simulink model "PFC_69C_03_06_V01_3Phase_3_2KW"  (R2022b)
settings: Solver=FixedStepAuto  StartTime=0.0  StopTime=Inf  RelTol=1e-3  EnableMultiTasking=on
model workspace (MAT data in the model file):
  ADC_Gain = 1241.21212121
  DAC_Gain = 0.000805860805861
  Inductor_Current_Divider_Gain_Phase_A = 33.4
  Inductor_Current_Divider_Gain_Phase_B = 33.4
  Vbulk_Divider_Gain = 276.854928018
  Vin_Divider_Gain = 556.17352614
undefined symbols (not defined in the file or in its folder): GPTRIP1SEL, GPTRIP2SEL, SCI_A_Transmit, SCI_A_Transmit_Current_Suffix, SCI_A_Transmit_one_shot_Suffix, SCI_A_Transmit_Polarity_Suffix, SCI_A_Transmit_relay_Suffix, SCI_A_Transmit_Vbulk_Suffix, SCI_A_Transmit_Vin_rms_Suffix, SCI_A_Transmit_Vin_Suffix, SCI_A_Transmit_Vmid_Suffix, SCI_A_Transmit_Vp_Suffix, SCI_A_Transmit_Vpfc_Suffix, TZ1, TZ2
libraries: c280xlib x38, c2802xlib x34, simulink x17, c2000lib x1
(part 6 of 8)

== system PFC_69C_03_06_V01_3Phase_3_2KW/Calibration,RMS, Fault Protection @5kHz/Fault checking/If Action Subsystem/Phase_C_Fault ==
  function : TriggerPort  TriggerType=function-call  VariantControl=(inherit)
  Fault Check (Input OVP)_Phase_C : Subsystem  TreatAsAtomicUnit=on
  Fault Check (Input UVP)_Phase_C : Subsystem  TreatAsAtomicUnit=on
  Function-Call Generator : simulink/Ports & Subsystems/Function-Call Generator  sample_time=-1  numberOfIterations=1  DisallowWideOutput=off
  Function-Call Split : FunctionCallSplit  IconShape=distinctive  NumOutputPorts=3  OutputPortLayout=default
  Input current_OCP_Phase_C : Subsystem  TreatAsAtomicUnit=on
  wires:
  Function-Call Generator/1 -> Function-Call Split/1
  Function-Call Split/1 -> Fault Check (Input UVP)_Phase_C/Trigger
  Function-Call Split/2 -> Fault Check (Input OVP)_Phase_C/Trigger
  Function-Call Split/3 -> Input current_OCP_Phase_C/Trigger

== system PFC_69C_03_06_V01_3Phase_3_2KW/Calibration,RMS, Fault Protection @5kHz/Polarity & Near Zero check/Polarity_Near_zero_Phase_A/Volt to Number ==
  In1 : Inport
  Gain : Gain  Gain=ADC_Gain
  Gain1 : Gain  Gain=1/Vin_Divider_Gain
  Out1 : Outport
  wires:
  Gain1/1 -> Gain/1
  In1/1 -> Gain1/1
  Gain/1 -> Out1/1

== system PFC_69C_03_06_V01_3Phase_3_2KW/Calibration,RMS, Fault Protection @5kHz/Polarity & Near Zero check/Polarity_Near_zero_Phase_B/Volt to Number ==
  In1 : Inport
  Gain : Gain  Gain=ADC_Gain
  Gain1 : Gain  Gain=1/Vin_Divider_Gain
  Out1 : Outport
  wires:
  Gain1/1 -> Gain/1
  In1/1 -> Gain1/1
  Gain/1 -> Out1/1

== system PFC_69C_03_06_V01_3Phase_3_2KW/Calibration,RMS, Fault Protection @5kHz/Polarity & Near Zero check/Polarity_Near_zero_Phase_C/Volt to Number ==
  In1 : Inport
  Gain : Gain  Gain=ADC_Gain
  Gain1 : Gain  Gain=1/Vin_Divider_Gain
  Out1 : Outport
  wires:
  Gain1/1 -> Gain/1
  In1/1 -> Gain1/1
  Gain/1 -> Out1/1

== system PFC_69C_03_06_V01_3Phase_3_2KW/Calibration,RMS, Fault Protection @5kHz/Relay control/Subsystem/ADC Gain2 ==
  In1 : Inport
  Gain : Gain  Gain=ADC_Gain
  Gain1 : Gain  Gain=1/Vin_Divider_Gain
  Out1 : Outport
  wires:
  Gain1/1 -> Gain/1
  In1/1 -> Gain1/1
  Gain/1 -> Out1/1

== system PFC_69C_03_06_V01_3Phase_3_2KW/Calibration,RMS, Fault Protection @5kHz/Relay control/Subsystem/ADC Gain3 ==
  In1 : Inport
  Gain : Gain  Gain=ADC_Gain
  Gain1 : Gain  Gain=1/Vin_Divider_Gain
  Out1 : Outport
  wires:
  Gain1/1 -> Gain/1
  In1/1 -> Gain1/1
  Gain/1 -> Out1/1

== system PFC_69C_03_06_V01_3Phase_3_2KW/Calibration,RMS, Fault Protection @5kHz/Relay control_corrected/Subsystem/ADC Gain2 ==
  In1 : Inport
  Gain : Gain  Gain=ADC_Gain
  Gain1 : Gain  Gain=1/Vin_Divider_Gain
  Out1 : Outport
  wires:
  Gain1/1 -> Gain/1
  In1/1 -> Gain1/1
  Gain/1 -> Out1/1

== system PFC_69C_03_06_V01_3Phase_3_2KW/Calibration,RMS, Fault Protection @5kHz/Relay control_corrected/Subsystem/ADC Gain3 ==
  In1 : Inport
  Gain : Gain  Gain=ADC_Gain
  Gain1 : Gain  Gain=1/Vin_Divider_Gain
  Out1 : Outport
  wires:
  Gain1/1 -> Gain/1
  In1/1 -> Gain1/1
  Gain/1 -> Out1/1

== system PFC_69C_03_06_V01_3Phase_3_2KW/Calibration,RMS, Fault Protection @5kHz/Voltage RMS//Averag Calculation/Phase_A/RMS Current Calculation_Phase_A ==
  note: RMS Voltage Calculation
  function : TriggerPort  TriggerType=function-call  VariantControl=(inherit)
  Chart : Stateflow chart  TreatAsAtomicUnit=on
  Data Store Read2 : DataStoreRead  DataStoreName=Inductor_Current_ADC_Phase_A  IndexOptions=Index vector (dialog)  Indices=1  OutputSizes=1
  Data Store Read5 : DataStoreRead  DataStoreName=Inductor_Current_1_65_ADC_Phase_A  IndexOptions=Index vector (dialog)  Indices=1  OutputSizes=1
  Data Store Write : DataStoreWrite  DataStoreName=Iin_rms_Phase_A  IndexOptions=Index vector (dialog)  Indices=1  OutputSizes=1
  Data Store Write1 : DataStoreWrite  DataStoreName=Iin_peak_Phase_A  IndexOptions=Index vector (dialog)  Indices=1  OutputSizes=1
  Gain1 : Gain  Gain=DAC_Gain
  Gain2 : Gain  Gain=DAC_Gain
  Gain3 : Gain  Gain=Inductor_Current_Divider_Gain_Phase_B
  Gain4 : Gain  Gain=Inductor_Current_Divider_Gain_Phase_B
  Gain5 : Gain  Gain=100
  Gain6 : Gain  Gain=100
  Subtract2 : Sum  Inputs=+-
  wires:
  Data Store Read2/1 -> Subtract2/1
  Data Store Read5/1 -> Subtract2/2
  Subtract2/1 -> Chart/1(input)
  Gain2/1 -> Gain3/1
  Chart/2(Vrms) -> Gain2/1
  Gain3/1 -> Gain6/1
  Gain6/1 -> Data Store Write/1
  Gain4/1 -> Gain5/1
  Gain1/1 -> Gain4/1
  Chart/1(Vpeak) -> Gain1/1
  Gain5/1 -> Data Store Write1/1

== system PFC_69C_03_06_V01_3Phase_3_2KW/Calibration,RMS, Fault Protection @5kHz/Voltage RMS//Averag Calculation/Phase_A/RMS Voltage Calculation_Phase_A ==
  note: RMS Voltage Calculation
  function : TriggerPort  TriggerType=function-call  VariantControl=(inherit)
  Chart : Stateflow chart  TreatAsAtomicUnit=on
  Data Store Read2 : DataStoreRead  DataStoreName=Vin_ADC_Average_Phase_A  IndexOptions=Index vector (dialog)  Indices=1  OutputSizes=1
  Data Store Read5 : DataStoreRead  DataStoreName=Vin_1_65_ADC_Phase_A  IndexOptions=Index vector (dialog)  Indices=1  OutputSizes=1
  Data Store Write1 : DataStoreWrite  DataStoreName=Vin_peak_Phase_A  IndexOptions=Index vector (dialog)  Indices=1  OutputSizes=1
  Data Store Write2 : DataStoreWrite  DataStoreName=Vin_rms_Phase_A  IndexOptions=Index vector (dialog)  Indices=1  OutputSizes=1
  Data Store Write3 : DataStoreWrite  DataStoreName=Vin_peak_ADC_Phase_A  IndexOptions=Index vector (dialog)  Indices=1  OutputSizes=1
  Data Store Write4 : DataStoreWrite  DataStoreName=Vin_rms_ADC  IndexOptions=Index vector (dialog)  Indices=1  OutputSizes=1
  Digital Output : c280xlib/Digital Output  Commented=on  GPIO_Number=GPIO16~GPIO23  GPIO_Bit0=off  GPIO_BIT0_Toggle=off  GPIO_Bit1=off  GPIO_BIT1_Toggle=off  GPIO_Bit2=off  GPIO_BIT2_Toggle=off  GPIO_Bit3=off  GPIO_BIT3_Toggle=off  GPIO_Bit4=off  GPIO_BIT4_Toggle=off  GPIO_Bit5=off  GPIO_BIT5_Toggle=off  GPIO_Bit6=on  GPIO_BIT6_Toggle=off  GPIO_Bit7=off  GPIO_BIT7_Toggle=off
  Gain6 : Gain  Gain=DAC_Gain
  Gain7 : Gain  Gain=Vin_Divider_Gain  OutDataTypeStr=double
  Gain8 : Gain  Gain=DAC_Gain
  Gain9 : Gain  Gain=Vin_Divider_Gain  OutDataTypeStr=double
  Subtract2 : Sum  Inputs=+-
  wires:
  Chart/1(Vpeak) -> Data Store Write3/1, Gain8/1
  Chart/2(Vrms) -> Gain6/1, Data Store Write4/1
  Gain7/1 -> Data Store Write2/1
  Data Store Read2/1 -> Subtract2/1
  Gain8/1 -> Gain9/1
  Gain6/1 -> Gain7/1
  Data Store Read5/1 -> Subtract2/2
  Gain9/1 -> Data Store Write1/1
  Subtract2/1 -> Chart/1(input)

== system PFC_69C_03_06_V01_3Phase_3_2KW/Calibration,RMS, Fault Protection @5kHz/Voltage RMS//Averag Calculation/Phase_A/Vin_ADC Averaging_Phase_A ==
  note: Low pass filter :
      | 1kHz bandwidth with 5kHz switching freq
  function : TriggerPort  TriggerType=function-call  VariantControl=(inherit)
  Chart1 : Stateflow chart  TreatAsAtomicUnit=on
  Constant1 : Constant  Value=0.38586954
  Constant2 : Constant  Value=0.38586954
  Constant3 : Constant  Value=-0.22826091
  Data Store Read3 : DataStoreRead  DataStoreName=Vin_ADC_Phase_A  IndexOptions=Index vector (dialog)  Indices=1  OutputSizes=1
  Vin_ADC_Average : DataStoreWrite  DataStoreName=Vin_ADC_Average_Phase_A  IndexOptions=Index vector (dialog)  Indices=1  OutputSizes=1
  wires:
  Constant3/1 -> [a1]
  Constant1/1 -> [b0]
  Constant2/1 -> [b1]
  [a1] -> Chart1/4(a1)
  [b1] -> Chart1/3(b1)
  [b0] -> Chart1/2(b0)
  Data Store Read3/1 -> Chart1/1(input_u)
  Chart1/1(output_y) -> Vin_ADC_Average/1

== system PFC_69C_03_06_V01_3Phase_3_2KW/Calibration,RMS, Fault Protection @5kHz/Voltage RMS//Averag Calculation/Phase_B/RMS Current Calculation_Phase_B ==
  note: RMS Voltage Calculation
  function : TriggerPort  TriggerType=function-call  VariantControl=(inherit)
  Chart : Stateflow chart  TreatAsAtomicUnit=on
  Data Store Read2 : DataStoreRead  DataStoreName=Inductor_Current_ADC_Phase_B  IndexOptions=Index vector (dialog)  Indices=1  OutputSizes=1
  Data Store Read5 : DataStoreRead  DataStoreName=Inductor_Current_1_65_ADC_Phase_B  IndexOptions=Index vector (dialog)  Indices=1  OutputSizes=1
  Data Store Write : DataStoreWrite  DataStoreName=Iin_rms_Phase_B  IndexOptions=Index vector (dialog)  Indices=1  OutputSizes=1
  Data Store Write1 : DataStoreWrite  DataStoreName=Iin_peak_Phase_B  IndexOptions=Index vector (dialog)  Indices=1  OutputSizes=1
  Gain1 : Gain  Gain=DAC_Gain
  Gain2 : Gain  Gain=DAC_Gain
  Gain3 : Gain  Gain=Inductor_Current_Divider_Gain_Phase_B
  Gain4 : Gain  Gain=Inductor_Current_Divider_Gain_Phase_B
  Gain5 : Gain  Gain=100
  Gain6 : Gain  Gain=100
  Subtract2 : Sum  Inputs=+-
  wires:
  Gain5/1 -> Data Store Write1/1
  Chart/1(Vpeak) -> Gain1/1
  Gain1/1 -> Gain4/1
  Gain4/1 -> Gain5/1
  Gain6/1 -> Data Store Write/1
  Gain3/1 -> Gain6/1
  Chart/2(Vrms) -> Gain2/1
  Gain2/1 -> Gain3/1
  Subtract2/1 -> Chart/1(input)
  Data Store Read5/1 -> Subtract2/2
  Data Store Read2/1 -> Subtract2/1

== system PFC_69C_03_06_V01_3Phase_3_2KW/Calibration,RMS, Fault Protection @5kHz/Voltage RMS//Averag Calculation/Phase_B/RMS Voltage Calculation_Phase_B ==
  note: RMS Voltage Calculation
  function : TriggerPort  TriggerType=function-call  VariantControl=(inherit)
  Chart : Stateflow chart  TreatAsAtomicUnit=on
  Data Store Read2 : DataStoreRead  DataStoreName=Vin_ADC_Average_Phase_B  IndexOptions=Index vector (dialog)  Indices=1  OutputSizes=1
  Data Store Read5 : DataStoreRead  DataStoreName=Vin_1_65_ADC_Phase_B  IndexOptions=Index vector (dialog)  Indices=1  OutputSizes=1
  Data Store Write1 : DataStoreWrite  DataStoreName=Vin_peak_Phase_B  IndexOptions=Index vector (dialog)  Indices=1  OutputSizes=1
  Data Store Write2 : DataStoreWrite  DataStoreName=Vin_rms_Phase_B  IndexOptions=Index vector (dialog)  Indices=1  OutputSizes=1
  Data Store Write3 : DataStoreWrite  DataStoreName=Vin_peak_ADC_Phase_B  IndexOptions=Index vector (dialog)  Indices=1  OutputSizes=1
  Data Store Write4 : DataStoreWrite  DataStoreName=Vin_rms_ADC  IndexOptions=Index vector (dialog)  Indices=1  OutputSizes=1
  Digital Output : c280xlib/Digital Output  Commented=on  GPIO_Number=GPIO16~GPIO23  GPIO_Bit0=off  GPIO_BIT0_Toggle=off  GPIO_Bit1=off  GPIO_BIT1_Toggle=off  GPIO_Bit2=off  GPIO_BIT2_Toggle=off  GPIO_Bit3=off  GPIO_BIT3_Toggle=off  GPIO_Bit4=off  GPIO_BIT4_Toggle=off  GPIO_Bit5=off  GPIO_BIT5_Toggle=off  GPIO_Bit6=on  GPIO_BIT6_Toggle=off  GPIO_Bit7=off  GPIO_BIT7_Toggle=off
  Gain6 : Gain  Gain=DAC_Gain
  Gain7 : Gain  Gain=Vin_Divider_Gain  OutDataTypeStr=double
  Gain8 : Gain  Gain=DAC_Gain
  Gain9 : Gain  Gain=Vin_Divider_Gain  OutDataTypeStr=double
  Subtract2 : Sum  Inputs=+-
  wires:
  Subtract2/1 -> Chart/1(input)
  Gain9/1 -> Data Store Write1/1
  Data Store Read5/1 -> Subtract2/2
  Gain6/1 -> Gain7/1
  Gain8/1 -> Gain9/1
  Data Store Read2/1 -> Subtract2/1
  Gain7/1 -> Data Store Write2/1
  Chart/2(Vrms) -> Data Store Write4/1, Gain6/1
  Chart/1(Vpeak) -> Gain8/1, Data Store Write3/1

== system PFC_69C_03_06_V01_3Phase_3_2KW/Calibration,RMS, Fault Protection @5kHz/Voltage RMS//Averag Calculation/Phase_B/Vin_ADC Averaging_Phase_B ==
  note: Low pass filter :
      | 1kHz bandwidth with 5kHz switching freq
  function : TriggerPort  TriggerType=function-call  VariantControl=(inherit)
  Chart1 : Stateflow chart  TreatAsAtomicUnit=on
  Constant1 : Constant  Value=0.38586954
  Constant2 : Constant  Value=0.38586954
  Constant3 : Constant  Value=-0.22826091
  Data Store Read3 : DataStoreRead  DataStoreName=Vin_ADC_Phase_B  IndexOptions=Index vector (dialog)  Indices=1  OutputSizes=1
  Vin_ADC_Average : DataStoreWrite  DataStoreName=Vin_ADC_Average_Phase_B  IndexOptions=Index vector (dialog)  Indices=1  OutputSizes=1
  wires:
  Chart1/1(output_y) -> Vin_ADC_Average/1
  Data Store Read3/1 -> Chart1/1(input_u)
  [b0] -> Chart1/2(b0)
  [b1] -> Chart1/3(b1)
  [a1] -> Chart1/4(a1)
  Constant2/1 -> [b1]
  Constant1/1 -> [b0]
  Constant3/1 -> [a1]

== system PFC_69C_03_06_V01_3Phase_3_2KW/Calibration,RMS, Fault Protection @5kHz/Voltage RMS//Averag Calculation/Phase_C/RMS Current Calculation_Phase_C ==
  note: RMS Voltage Calculation
  function : TriggerPort  TriggerType=function-call  VariantControl=(inherit)
  Chart : Stateflow chart  TreatAsAtomicUnit=on
  Data Store Read2 : DataStoreRead  DataStoreName=Inductor_Current_ADC_Phase_C  IndexOptions=Index vector (dialog)  Indices=1  OutputSizes=1
  Data Store Read5 : DataStoreRead  DataStoreName=Inductor_Current_1_65_ADC_Phase_C  IndexOptions=Index vector (dialog)  Indices=1  OutputSizes=1
  Data Store Write : DataStoreWrite  DataStoreName=Iin_rms_Phase_C  IndexOptions=Index vector (dialog)  Indices=1  OutputSizes=1
  Data Store Write1 : DataStoreWrite  DataStoreName=Iin_peak_Phase_C  IndexOptions=Index vector (dialog)  Indices=1  OutputSizes=1
  Gain1 : Gain  Gain=DAC_Gain
  Gain2 : Gain  Gain=DAC_Gain
  Gain3 : Gain  Gain=Inductor_Current_Divider_Gain_Phase_B
  Gain4 : Gain  Gain=Inductor_Current_Divider_Gain_Phase_B
  Gain5 : Gain  Gain=100
  Gain6 : Gain  Gain=100
  Subtract2 : Sum  Inputs=+-
  wires:
  Data Store Read2/1 -> Subtract2/1
  Data Store Read5/1 -> Subtract2/2
  Subtract2/1 -> Chart/1(input)
  Gain2/1 -> Gain3/1
  Chart/2(Vrms) -> Gain2/1
  Gain3/1 -> Gain6/1
  Gain6/1 -> Data Store Write/1
  Gain5/1 -> Data Store Write1/1
  Gain1/1 -> Gain4/1
  Gain4/1 -> Gain5/1
  Chart/1(Vpeak) -> Gain1/1

== system PFC_69C_03_06_V01_3Phase_3_2KW/Calibration,RMS, Fault Protection @5kHz/Voltage RMS//Averag Calculation/Phase_C/RMS Voltage Calculation_Phase_C ==
  note: RMS Voltage Calculation
  function : TriggerPort  TriggerType=function-call  VariantControl=(inherit)
  Chart : Stateflow chart  TreatAsAtomicUnit=on
  Data Store Read2 : DataStoreRead  DataStoreName=Vin_ADC_Average_Phase_C  IndexOptions=Index vector (dialog)  Indices=1  OutputSizes=1
  Data Store Read5 : DataStoreRead  DataStoreName=Vin_1_65_ADC_Phase_C  IndexOptions=Index vector (dialog)  Indices=1  OutputSizes=1
  Data Store Write1 : DataStoreWrite  DataStoreName=Vin_peak_Phase_C  IndexOptions=Index vector (dialog)  Indices=1  OutputSizes=1
  Data Store Write2 : DataStoreWrite  DataStoreName=Vin_rms_Phase_C  IndexOptions=Index vector (dialog)  Indices=1  OutputSizes=1
  Data Store Write3 : DataStoreWrite  DataStoreName=Vin_peak_ADC_Phase_C  IndexOptions=Index vector (dialog)  Indices=1  OutputSizes=1
  Data Store Write4 : DataStoreWrite  DataStoreName=Vin_rms_ADC  IndexOptions=Index vector (dialog)  Indices=1  OutputSizes=1
  Gain6 : Gain  Gain=DAC_Gain
  Gain7 : Gain  Gain=Vin_Divider_Gain  OutDataTypeStr=double
  Gain8 : Gain  Gain=DAC_Gain
  Gain9 : Gain  Gain=Vin_Divider_Gain  OutDataTypeStr=double
  Subtract2 : Sum  Inputs=+-
  wires:
  Chart/1(Vpeak) -> Data Store Write3/1, Gain8/1
  Chart/2(Vrms) -> Gain6/1, Data Store Write4/1
  Gain7/1 -> Data Store Write2/1
  Data Store Read2/1 -> Subtract2/1
  Gain8/1 -> Gain9/1
  Gain6/1 -> Gain7/1
  Data Store Read5/1 -> Subtract2/2
  Gain9/1 -> Data Store Write1/1
  Subtract2/1 -> Chart/1(input)

== system PFC_69C_03_06_V01_3Phase_3_2KW/Calibration,RMS, Fault Protection @5kHz/Voltage RMS//Averag Calculation/Phase_C/Vin_ADC Averaging_Phase_C ==
  note: Low pass filter :
      | 1kHz bandwidth with 5kHz switching freq
  function : TriggerPort  TriggerType=function-call  VariantControl=(inherit)
  Chart1 : Stateflow chart  TreatAsAtomicUnit=on
  Constant1 : Constant  Value=0.38586954
  Constant2 : Constant  Value=0.38586954
  Constant3 : Constant  Value=-0.22826091
  Data Store Read3 : DataStoreRead  DataStoreName=Vin_ADC_Phase_C  IndexOptions=Index vector (dialog)  Indices=1  OutputSizes=1
  Vin_ADC_Average : DataStoreWrite  DataStoreName=Vin_ADC_Average_Phase_C  IndexOptions=Index vector (dialog)  Indices=1  OutputSizes=1
  wires:
  Constant3/1 -> [a1]
  Constant1/1 -> [b0]
  Constant2/1 -> [b1]
  [a1] -> Chart1/4(a1)
  [b1] -> Chart1/3(b1)
  [b0] -> Chart1/2(b0)
  Data Store Read3/1 -> Chart1/1(input_u)
  Chart1/1(output_y) -> Vin_ADC_Average/1

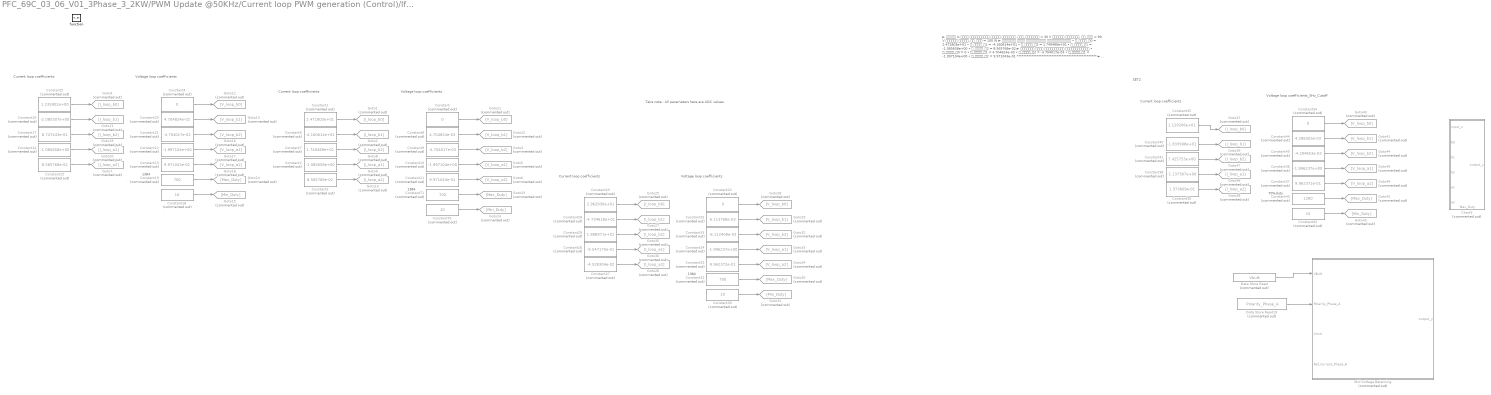
== system PFC_69C_03_06_V01_3Phase_3_2KW/PWM Update @50KHz/Current loop PWM generation (Control)/If Action Subsystem/Function-Call Subsystem ==
  note: Take note : All parameters here are ADC values.
  note: ► 𝑷𝒍𝒂𝒏𝒕 & 𝑳𝒐𝒂𝒅 𝒑𝒂𝒓𝒂𝒎𝒆𝒕𝒆𝒓𝒔
      | 𝑰𝒏𝒑𝒖𝒕 𝒗𝒐𝒍𝒕𝒂𝒈𝒆, 𝑽𝒊𝒏_𝒏𝒐𝒎𝒊𝒏𝒂𝒍 = 30 V
      | 𝑶𝒖𝒕𝒑𝒖𝒕 𝒗𝒐𝒍𝒕𝒂𝒈𝒆, 𝑽𝒐_𝑷𝑭𝑪 = 90 V
      | 𝑶𝒖𝒕𝒑𝒖𝒕 𝒑𝒐𝒘𝒆𝒓, 𝑷𝒐_𝑷𝑭𝑪 = 100 W
      |
      | ► 𝑪𝒖𝒓𝒓𝒆𝒏𝒕 𝒍𝒐𝒐𝒑 𝒄𝒐𝒏𝒕𝒓𝒐𝒍𝒍𝒆𝒓 𝒄𝒐𝒆𝒇𝒇𝒊𝒄𝒊𝒆𝒏𝒕𝒔
      | • 𝑰_𝒍𝒐𝒐𝒑_𝒃0 = 2.471803e+01
      | • 𝑰_𝒍𝒐𝒐𝒑_𝒃1 = -4.160614e+01
      | • 𝑰_𝒍𝒐𝒐𝒑_𝒃2 = 1.749489e+01
      | • 𝑰_𝒍𝒐𝒐𝒑_𝒂1 = -1.085658e+00
      | • 𝑰_𝒍𝒐𝒐𝒑_𝒂2 = 8.565768e-02
      |
      | ► 𝑽𝒐𝒍𝒕𝒂𝒈𝒆 𝒍𝒐𝒐𝒑 𝒄𝒐𝒏𝒕𝒓𝒐𝒍𝒍𝒆𝒓 𝒄𝒐𝒆𝒇𝒇𝒊𝒄𝒊𝒆𝒏𝒕𝒔
      | • 𝑽_𝒍𝒐𝒐𝒑_𝒃0 = 0
      | • 𝑽_𝒍𝒐𝒐𝒑_𝒃1 = 4.704824e-03
      | • 𝑽_𝒍𝒐𝒐𝒑_𝒃2 = -4.704017e-03
      | • 𝑽_𝒍𝒐𝒐𝒑_𝒂1 = -1.997104e+00
      | • 𝑽_𝒍𝒐𝒐𝒑_𝒂2 = 9.971043e-01
      |
      | ************************************************
      | ► 𝑻𝒉𝒆 𝒇𝒐𝒓𝒎𝒂𝒕 𝒇𝒐𝒓 𝒄𝒐𝒆𝒇𝒇𝒊𝒄𝒊𝒆𝒏𝒕𝒔 𝒊𝒔 𝒔𝒉𝒐𝒘𝒏 𝒃𝒆𝒍𝒐𝒘.
      |
      | 𝒚(𝒌) = 𝒃0 𝒆(𝒌) + 𝒃1 𝒆(𝒌−1) + 𝒃2 𝒆(𝒌−2) − 𝒂1 𝒚(𝒌−1) − 𝒂2 𝒚(𝒌−2)
      |
      | ************************************************
      | ◘◘◘◘◘◘◘◘◘◘◘◘◘◘◘◘◘◘◘◘◘◘◘◘◘◘◘◘◘◘◘◘◘◘◘◘◘◘◘◘◘◘◘◘◘◘◘◘
  note: Current loop coefficients
  note: Voltage loop coefficients
  note: 1384
  note: Current loop coefficients
  note: Current loop coefficients
  note: SET2
  note: Voltage loop coefficients
  note: 1384
  note: Voltage loop coefficients_5Hz_Cutoff
  note: 70%duty
  note: Voltage loop coefficients
  note: 1384
  note: Current loop coefficients
  function : TriggerPort  TriggerType=function-call  VariantControl=(inherit)
  Chart3 : Stateflow chart  Commented=on  TreatAsAtomicUnit=on
      settings: PortSchema="{\"entries\":[{\"content\":{\"sides\":[{\"content\":{\"connectorIds\":[\"In2\",\"In3\",\"In4\",\"In5\",\"In6\",\"In7\"]},\"type\":\"ConnectorPlacement.EquallySpacedRectSide\",\"uuid\":\"98054acb-dc05-45b7-9e49-d1f1309a60af\"},{\"content\":{\"connectorIds\":[\"Out1\"],\"side\":\"RIGHT\"},\"type\":\"ConnectorPlacement.EquallySpacedRectSide\",\"uuid\":\"519c6a11-fba4-4420-9bc2-f24cec898983\"},{\"content\":{\"connectorIds\":[],\"side\":\"TOP\"},\"type\":\"ConnectorPlacement.EquallySpacedRectSide\",\"uuid\":\"37e92206-8070-4c6c-85b3-8eb12c5538cd\"},{\"content\":{\"connectorIds\":[\"In1\"],\"side\":\"BOTTOM\"},\"type\":\"ConnectorPlacement.EquallySpacedRectSide\",\"uuid\":\"2f414d73-99cb-441b-a85c-e16df8718e53\"}]},\"type\":\"ConnectorPlacement.EquallySpacedConnector\",\"uuid\":\"7d467722-ac20-43d4-98e5-7341f60d2894\"}],\"packageUris\":[\"http://schema.mathworks.com/mf0/Connector/R2020b\"],\"version\":\"1.0\"}"
  Constant{,4,22,34} (4 alike) : Constant  Commented=on  Value=0
  Constant1 : Constant  Commented=on  Value=2.471803e+01
  Constant10 : Constant  Commented=on  Value=-1.997104e+00
  Constant11 : Constant  Commented=on  Value=9.971043e-01
  Constant12 : Constant  Commented=on  Value=-1.997104e+00
  Constant13 : Constant  Commented=on  Value=9.971043e-01
  Constant14 : Constant  Commented=on  Value=-1.085658e+00
  Constant15 : Constant  Commented=on  Value=8.565768e-02
  Constant16 : Constant  Commented=on  Value=-2.080307e+00
  Constant17 : Constant  Commented=on  Value=8.747443e-01
  Constant{18,30,42,70} (4 alike) : Constant  Commented=on  Value=10  OutDataTypeStr=double
  Constant19 : Constant  Commented=on  Value=700  OutDataTypeStr=double
  Constant2 : Constant  Commented=on  Value=-1.085658e+00
  Constant20 : Constant  Commented=on  Value=4.704824e-02
  Constant21 : Constant  Commented=on  Value=-4.704017e-02
  Constant23 : Constant  Commented=on  Value=2.962930e+01
  Constant24 : Constant  Commented=on  Value=-1.996237e+00
  Constant25 : Constant  Commented=on  Value=9.962372e-01
  Constant26 : Constant  Commented=on  Value=-9.547170e-01
  Constant27 : Constant  Commented=on  Value=-4.528304e-02
  Constant28 : Constant  Commented=on  Value=-4.734618e+01
  Constant29 : Constant  Commented=on  Value=1.888971e+01
  Constant3 : Constant  Commented=on  Value=8.565768e-02
  Constant31 : Constant  Commented=on  Value=700  OutDataTypeStr=double
  Constant32 : Constant  Commented=on  Value=6.113768e-03
  Constant33 : Constant  Commented=on  Value=-6.112408e-03
  Constant35 : Constant  Commented=on  Value=1.129206e+01
  Constant36 : Constant  Commented=on  Value=-1.996237e+00
  Constant37 : Constant  Commented=on  Value=9.962372e-01
  Constant38 : Constant  Commented=on  Value=-1.137367e+00
  Constant39 : Constant  Commented=on  Value=1.373669e-01
  Constant40 : Constant  Commented=on  Value=-1.833908e+01
  Constant41 : Constant  Commented=on  Value=7.425753e+00
  Constant43 : Constant  Commented=on  Value=1260  OutDataTypeStr=double
  Constant44 : Constant  Commented=on  Value=4.286303e-03
  Constant45 : Constant  Commented=on  Value=-4.284853e-03
  Constant5 : Constant  Commented=on  Value=1.235902e+00
  Constant6 : Constant  Commented=on  Value=-4.160614e+01
  Constant7 : Constant  Commented=on  Value=1.749489e+01
  Constant71 : Constant  Commented=on  Value=700  OutDataTypeStr=double
  Constant8 : Constant  Commented=on  Value=4.704824e-03
  Constant9 : Constant  Commented=on  Value=-4.704017e-03
  Data Store Read : DataStoreRead  Commented=on  DataStoreName=Vbulk  IndexOptions=Index vector (dialog)  Indices=1  OutputSizes=1
  Data Store Read19 : DataStoreRead  Commented=on  DataStoreName=Polarity_Phase_A  IndexOptions=Index vector (dialog)  Indices=1  OutputSizes=1
  Goto{1,4,25,37} (4 alike) : Goto  Commented=on  GotoTag=I_loop_b0
  Goto{7,10,26,38} (4 alike) : Goto  Commented=on  GotoTag=I_loop_a2
  Goto{2,11,27,39} (4 alike) : Goto  Commented=on  GotoTag=I_loop_b1
  Goto{12,21,28,40} (4 alike) : Goto  Commented=on  GotoTag=V_loop_b0
  Goto{13,22,29,41} (4 alike) : Goto  Commented=on  GotoTag=V_loop_b1
  Goto{14,23,30,42} (4 alike) : Goto  Commented=on  GotoTag=Max_Duty
  Goto{15,24,31,43} (4 alike) : Goto  Commented=on  GotoTag=Min_Duty
  Goto{3,16,32,44} (4 alike) : Goto  Commented=on  GotoTag=V_loop_b2
  Goto{5,17,33,45} (4 alike) : Goto  Commented=on  GotoTag=V_loop_a1
  Goto{6,18,34,46} (4 alike) : Goto  Commented=on  GotoTag=V_loop_a2
  Goto{8,19,35,47} (4 alike) : Goto  Commented=on  GotoTag=I_loop_b2
  Goto{9,20,36,48} (4 alike) : Goto  Commented=on  GotoTag=I_loop_a1
  Mid Voltage Balancing : Stateflow chart  Commented=on  TreatAsAtomicUnit=on
  wires:
  Constant14/1 -> Goto20/1
  Constant29/1 -> Goto35/1
  Constant30/1 -> Goto31/1
  Constant35/1 -> Goto37/1
  Constant43/1 -> Goto42/1
  Data Store Read/1 -> Mid Voltage Balancing/1(VBulk)
  Data Store Read19/1 -> Mid Voltage Balancing/2(Polarity_Phase_A)
  Constant37/1 -> Goto46/1
  Constant/1 -> Goto21/1
  Constant45/1 -> Goto44/1
  Constant15/1 -> Goto7/1
  Constant42/1 -> Goto43/1
  Constant18/1 -> Goto15/1
  Constant71/1 -> Goto23/1
  Constant41/1 -> Goto47/1
  Constant31/1 -> Goto30/1
  Constant40/1 -> Goto39/1
  Constant12/1 -> Goto17/1
  Constant44/1 -> Goto41/1
  Constant39/1 -> Goto38/1
  Constant22/1 -> Goto28/1
  Constant28/1 -> Goto27/1
  Constant8/1 -> Goto22/1
  Constant19/1 -> Goto14/1
  Constant34/1 -> Goto40/1
  Constant36/1 -> Goto45/1
  Constant23/1 -> Goto25/1
  Constant25/1 -> Goto34/1
  Constant38/1 -> Goto48/1
  Constant20/1 -> Goto13/1
  Constant26/1 -> Goto36/1
  Constant5/1 -> Goto4/1
  Constant16/1 -> Goto11/1
  Constant17/1 -> Goto19/1
  Constant9/1 -> Goto3/1
  Constant24/1 -> Goto33/1
  Constant10/1 -> Goto5/1
  Constant27/1 -> Goto26/1
  Constant7/1 -> Goto8/1
  Constant6/1 -> Goto2/1
  Constant21/1 -> Goto16/1
  Constant3/1 -> Goto10/1
  Constant4/1 -> Goto12/1
  Constant1/1 -> Goto1/1
  Constant70/1 -> Goto24/1
  Constant2/1 -> Goto9/1
  Constant13/1 -> Goto18/1
  Constant11/1 -> Goto6/1
  Constant33/1 -> Goto32/1
  Constant32/1 -> Goto29/1
  ? -> Mid Voltage Balancing/3(Vmid)

== system PFC_69C_03_06_V01_3Phase_3_2KW/PWM Update @50KHz/Fixed Duty update_Phase_A/Archive/If Action Subsystem ==
  Action Port : ActionPort  ActionPortLabel=if(u1 ==0)
  Constant : Constant  Value=0
  Data Store Write : DataStoreWrite  DataStoreName=PWM_DutyNearzero  IndexOptions=Index vector (dialog)  Indices=1  OutputSizes=1
  wires:
  Constant/1 -> Data Store Write/1

== system PFC_69C_03_06_V01_3Phase_3_2KW/PWM Update @50KHz/Fixed Duty update_Phase_A/Archive/If Action Subsystem1 ==
  In1 : Inport  OutDataTypeStr=double
  Action Port : ActionPort  ActionPortLabel=if(u1 ==1)
  Out1 : Outport  OutDataTypeStr=double
  wires:
  In1/1 -> Out1/1

== system PFC_69C_03_06_V01_3Phase_3_2KW/PWM Update @50KHz/Fixed Duty update_Phase_A/Archive/If Action Subsystem2 ==
  In1 : Inport
  Action Port : ActionPort  ActionPortLabel=else
  Out1 : Outport
  wires:
  In1/1 -> Out1/1

== system PFC_69C_03_06_V01_3Phase_3_2KW/PWM Update @50KHz/Fixed Duty update_Phase_A/Archive/If Action Subsystem3 ==
  Action Port : ActionPort  ActionPortLabel=else
  Data Store Read7 : DataStoreRead  DataStoreName=Polarity_Phase_A  IndexOptions=Index vector (dialog)  Indices=1  OutputSizes=1
  If Action Subsystem4 : Subsystem  TreatAsAtomicUnit=on
  If Action Subsystem5 : Subsystem  TreatAsAtomicUnit=on
  If2 : If  IfExpression=u1 ==1
  wires:
  Data Store Read7/1 -> If2/1
  If2/2 -> If Action Subsystem5/Action
  If2/1 -> If Action Subsystem4/Action

== system PFC_69C_03_06_V01_3Phase_3_2KW/PWM Update @50KHz/Fixed Duty update_Phase_B_Test/Archive/If Action Subsystem ==
  Action Port : ActionPort
  Constant : Constant  Value=0
  Data Store Write : DataStoreWrite  DataStoreName=PWM_DutyNearzero  IndexOptions=Index vector (dialog)  Indices=1  OutputSizes=1
  wires:
  Constant/1 -> Data Store Write/1

== system PFC_69C_03_06_V01_3Phase_3_2KW/PWM Update @50KHz/Fixed Duty update_Phase_B_Test/Archive/If Action Subsystem1 ==
  In1 : Inport  OutDataTypeStr=double
  Action Port : ActionPort
  Out1 : Outport  OutDataTypeStr=double
  wires:
  In1/1 -> Out1/1

== system PFC_69C_03_06_V01_3Phase_3_2KW/PWM Update @50KHz/Fixed Duty update_Phase_B_Test/Archive/If Action Subsystem2 ==
  In1 : Inport
  Action Port : ActionPort
  Out1 : Outport
  wires:
  In1/1 -> Out1/1

== system PFC_69C_03_06_V01_3Phase_3_2KW/PWM Update @50KHz/Fixed Duty update_Phase_B_Test/Archive/If Action Subsystem3 ==
  Action Port : ActionPort
  Data Store Read7 : DataStoreRead  DataStoreName=Polarity_Phase_A  IndexOptions=Index vector (dialog)  Indices=1  OutputSizes=1
  If Action Subsystem4 : Subsystem  TreatAsAtomicUnit=on
  If Action Subsystem5 : Subsystem  TreatAsAtomicUnit=on
  If2 : If  IfExpression=u1 ==1
  wires:
  Data Store Read7/1 -> If2/1
  If2/2 -> If Action Subsystem5/Action
  If2/1 -> If Action Subsystem4/Action

== system PFC_69C_03_06_V01_3Phase_3_2KW/PWM Update @50KHz/Fixed Duty update_Phase_C/Archive/If Action Subsystem ==
  Action Port : ActionPort
  Constant : Constant  Value=0
  Data Store Write : DataStoreWrite  DataStoreName=PWM_DutyNearzero  IndexOptions=Index vector (dialog)  Indices=1  OutputSizes=1
  wires:
  Constant/1 -> Data Store Write/1

== system PFC_69C_03_06_V01_3Phase_3_2KW/PWM Update @50KHz/Fixed Duty update_Phase_C/Archive/If Action Subsystem1 ==
  In1 : Inport  OutDataTypeStr=double
  Action Port : ActionPort
  Out1 : Outport  OutDataTypeStr=double
  wires:
  In1/1 -> Out1/1

== system PFC_69C_03_06_V01_3Phase_3_2KW/PWM Update @50KHz/Fixed Duty update_Phase_C/Archive/If Action Subsystem2 ==
  In1 : Inport
  Action Port : ActionPort
  Out1 : Outport
  wires:
  In1/1 -> Out1/1

== system PFC_69C_03_06_V01_3Phase_3_2KW/PWM Update @50KHz/Fixed Duty update_Phase_C/Archive/If Action Subsystem3 ==
  Action Port : ActionPort
  Data Store Read7 : DataStoreRead  DataStoreName=Polarity_Phase_A  IndexOptions=Index vector (dialog)  Indices=1  OutputSizes=1
  If Action Subsystem4 : Subsystem  TreatAsAtomicUnit=on
  If Action Subsystem5 : Subsystem  TreatAsAtomicUnit=on
  If2 : If  IfExpression=u1 ==1
  wires:
  Data Store Read7/1 -> If2/1
  If2/2 -> If Action Subsystem5/Action
  If2/1 -> If Action Subsystem4/Action

== system PFC_69C_03_06_V01_3Phase_3_2KW/Calibration,RMS, Fault Protection @5kHz/Fault checking/If Action Subsystem/Phase_A_Fault/Fault Check (Input OVP)_Phase_A  ==
  note: "Von_Threshold" is set inside this state machine
  note: Fault Check (Input UVP)
  function : TriggerPort  TriggerType=function-call  VariantControl=(inherit)
  Chart1 : Stateflow chart  TreatAsAtomicUnit=on
  Data Store Read3 : DataStoreRead  DataStoreName=Vin_rms_Phase_A  IndexOptions=Index vector (dialog)  Indices=1  OutputSizes=1
  Data Store Write : DataStoreWrite  DataStoreName=Vin_OVP_Flag_Phase_A  IndexOptions=Index vector (dialog)  Indices=1  OutputSizes=1
  wires:
  Data Store Read3/1 -> Chart1/1(input)
  Chart1/1(Input_OVP_Flag) -> Data Store Write/1

== system PFC_69C_03_06_V01_3Phase_3_2KW/Calibration,RMS, Fault Protection @5kHz/Fault checking/If Action Subsystem/Phase_A_Fault/Fault Check (Input UVP)_Phase_A  ==
  note: "Von_Threshold" is set inside this state machine
  note: Fault Check (Input UVP)
  function : TriggerPort  TriggerType=function-call  VariantControl=(inherit)
  Chart1 : Stateflow chart  TreatAsAtomicUnit=on
  Data Store Read3 : DataStoreRead  DataStoreName=Vin_rms_Phase_A  IndexOptions=Index vector (dialog)  Indices=1  OutputSizes=1
  Data Store Write : DataStoreWrite  DataStoreName=Vin_UVP_Flag_Phase_A  IndexOptions=Index vector (dialog)  Indices=1  OutputSizes=1
  wires:
  Data Store Read3/1 -> Chart1/1(input)
  Chart1/1(Input_UVP_Flag) -> Data Store Write/1

== system PFC_69C_03_06_V01_3Phase_3_2KW/Calibration,RMS, Fault Protection @5kHz/Fault checking/If Action Subsystem/Phase_A_Fault/Input current_OCP_Phase_A ==
  note: Vbulk_OVP_Threshold initialized in Data Store Memory
  note: Output Voltage_Latch_OVP
  function : TriggerPort  TriggerType=function-call  VariantControl=(inherit)
  Abs : Abs  SaturateOnIntegerOverflow=off
  Chart2 : Stateflow chart  TreatAsAtomicUnit=on
  Data Store Read : DataStoreRead  DataStoreName=Inductor_Current_ADC_Phase_A  IndexOptions=Index vector (dialog)  Indices=1  OutputSizes=1
  Data Store Read1 : DataStoreRead  DataStoreName=Iin_OCP_Threshold  IndexOptions=Index vector (dialog)  Indices=1  OutputSizes=1
  Data Store Read3 : DataStoreRead  DataStoreName=Inductor_Current_1_65_ADC_Phase_A  IndexOptions=Index vector (dialog)  Indices=1  OutputSizes=1
  Data Store Write1 : DataStoreWrite  DataStoreName=Iin_OCP_Flag_phase_A  IndexOptions=Index vector (dialog)  Indices=1  OutputSizes=1
  Gain2 : Gain  Gain=0.00080586
  Gain3 : Gain  Gain=33.445
  Subtract2 : Sum  Inputs=+-
  wires:
  Gain3/1 -> Abs/1
  Data Store Read3/1 -> Subtract2/2
  Data Store Read/1 -> Subtract2/1
  Chart2/1(Iin_OCP_Flag) -> Data Store Write1/1
  Gain2/1 -> Gain3/1
  Subtract2/1 -> Gain2/1
  Abs/1 -> Chart2/1(input_Iin)
  Data Store Read1/1 -> Chart2/2("OCP_Threshold ")

== system PFC_69C_03_06_V01_3Phase_3_2KW/Calibration,RMS, Fault Protection @5kHz/Fault checking/If Action Subsystem/Phase_B_Fault/Fault Check (Input OVP)_Phase_B ==
  note: "Von_Threshold" is set inside this state machine
  note: Fault Check (Input UVP)
  function : TriggerPort  TriggerType=function-call  VariantControl=(inherit)
  Chart1 : Stateflow chart  TreatAsAtomicUnit=on
  Data Store Read3 : DataStoreRead  DataStoreName=Vin_rms_Phase_B  IndexOptions=Index vector (dialog)  Indices=1  OutputSizes=1
  Data Store Write : DataStoreWrite  DataStoreName=Vin_OVP_Flag_Phase_B  IndexOptions=Index vector (dialog)  Indices=1  OutputSizes=1
  wires:
  Data Store Read3/1 -> Chart1/1(input)
  Chart1/1(Input_OVP_Flag) -> Data Store Write/1

== system PFC_69C_03_06_V01_3Phase_3_2KW/Calibration,RMS, Fault Protection @5kHz/Fault checking/If Action Subsystem/Phase_B_Fault/Fault Check (Input UVP)_Phase_B ==
  note: "Von_Threshold" is set inside this state machine
  note: Fault Check (Input UVP)
  function : TriggerPort  TriggerType=function-call  VariantControl=(inherit)
  Chart1 : Stateflow chart  TreatAsAtomicUnit=on
  Data Store Read3 : DataStoreRead  DataStoreName=Vin_rms_Phase_B  IndexOptions=Index vector (dialog)  Indices=1  OutputSizes=1
  Data Store Write : DataStoreWrite  DataStoreName=Vin_UVP_Flag_Phase_B  IndexOptions=Index vector (dialog)  Indices=1  OutputSizes=1
  wires:
  Data Store Read3/1 -> Chart1/1(input)
  Chart1/1(Input_UVP_Flag) -> Data Store Write/1

== system PFC_69C_03_06_V01_3Phase_3_2KW/Calibration,RMS, Fault Protection @5kHz/Fault checking/If Action Subsystem/Phase_B_Fault/Input current_OCP_Phase_B ==
  note: Output Voltage_Latch_OVP
  function : TriggerPort  TriggerType=function-call  VariantControl=(inherit)
  Abs : Abs  SaturateOnIntegerOverflow=off
  Chart2 : Stateflow chart  TreatAsAtomicUnit=on
  Data Store Read : DataStoreRead  DataStoreName=Inductor_Current_ADC_Phase_B  IndexOptions=Index vector (dialog)  Indices=1  OutputSizes=1
  Data Store Read1 : DataStoreRead  DataStoreName=Iin_OCP_Threshold  IndexOptions=Index vector (dialog)  Indices=1  OutputSizes=1
  Data Store Read3 : DataStoreRead  DataStoreName=Inductor_Current_1_65_ADC_Phase_B  IndexOptions=Index vector (dialog)  Indices=1  OutputSizes=1
  Data Store Write1 : DataStoreWrite  DataStoreName=Iin_OCP_Flag_phase_B  IndexOptions=Index vector (dialog)  Indices=1  OutputSizes=1
  Gain2 : Gain  Gain=0.00080586
  Gain3 : Gain  Gain=33.445
  Subtract2 : Sum  Inputs=+-
  wires:
  Data Store Read3/1 -> Subtract2/2
  Subtract2/1 -> Gain2/1
  Data Store Read/1 -> Subtract2/1
  Abs/1 -> Chart2/1(input_Iin)
  Chart2/1(Iin_OCP_Flag) -> Data Store Write1/1
  Data Store Read1/1 -> Chart2/2("OCP_Threshold ")
  Gain2/1 -> Gain3/1
  Gain3/1 -> Abs/1

== system PFC_69C_03_06_V01_3Phase_3_2KW/Calibration,RMS, Fault Protection @5kHz/Fault checking/If Action Subsystem/Phase_C_Fault/Fault Check (Input OVP)_Phase_C ==
  note: "Von_Threshold" is set inside this state machine
  note: Fault Check (Input UVP)
  function : TriggerPort  TriggerType=function-call  VariantControl=(inherit)
  Chart1 : Stateflow chart  TreatAsAtomicUnit=on
  Data Store Read3 : DataStoreRead  DataStoreName=Vin_rms_Phase_C  IndexOptions=Index vector (dialog)  Indices=1  OutputSizes=1
  Data Store Write : DataStoreWrite  DataStoreName=Vin_OVP_Flag_Phase_C  IndexOptions=Index vector (dialog)  Indices=1  OutputSizes=1
  wires:
  Data Store Read3/1 -> Chart1/1(input)
  Chart1/1(Input_OVP_Flag) -> Data Store Write/1

== system PFC_69C_03_06_V01_3Phase_3_2KW/Calibration,RMS, Fault Protection @5kHz/Fault checking/If Action Subsystem/Phase_C_Fault/Fault Check (Input UVP)_Phase_C ==
  note: "Von_Threshold" is set inside this state machine
  note: Fault Check (Input UVP)
  function : TriggerPort  TriggerType=function-call  VariantControl=(inherit)
  Chart1 : Stateflow chart  TreatAsAtomicUnit=on
  Data Store Read3 : DataStoreRead  DataStoreName=Vin_rms_Phase_C  IndexOptions=Index vector (dialog)  Indices=1  OutputSizes=1
  Data Store Write : DataStoreWrite  DataStoreName=Vin_UVP_Flag_Phase_C  IndexOptions=Index vector (dialog)  Indices=1  OutputSizes=1
  wires:
  Data Store Read3/1 -> Chart1/1(input)
  Chart1/1(Input_UVP_Flag) -> Data Store Write/1

== system PFC_69C_03_06_V01_3Phase_3_2KW/Calibration,RMS, Fault Protection @5kHz/Fault checking/If Action Subsystem/Phase_C_Fault/Input current_OCP_Phase_C ==
  note: Output Voltage_Latch_OVP
  note: Vbulk_OVP_Threshold initialized in Data Store Memory
  function : TriggerPort  TriggerType=function-call  VariantControl=(inherit)
  Abs : Abs  SaturateOnIntegerOverflow=off
  Chart2 : Stateflow chart  TreatAsAtomicUnit=on
  Data Store Read : DataStoreRead  DataStoreName=Inductor_Current_ADC_Phase_C  IndexOptions=Index vector (dialog)  Indices=1  OutputSizes=1
  Data Store Read1 : DataStoreRead  DataStoreName=Iin_OCP_Threshold  IndexOptions=Index vector (dialog)  Indices=1  OutputSizes=1
  Data Store Read3 : DataStoreRead  DataStoreName=Inductor_Current_1_65_ADC_Phase_C  IndexOptions=Index vector (dialog)  Indices=1  OutputSizes=1
  Data Store Write1 : DataStoreWrite  DataStoreName=Iin_OCP_Flag_phase_C  IndexOptions=Index vector (dialog)  Indices=1  OutputSizes=1
  Gain2 : Gain  Gain=0.00080586
  Gain3 : Gain  Gain=33.445
  Subtract2 : Sum  Inputs=+-
  wires:
  Data Store Read3/1 -> Subtract2/2
  Subtract2/1 -> Gain2/1
  Data Store Read/1 -> Subtract2/1
  Abs/1 -> Chart2/1(input_Iin)
  Chart2/1(Iin_OCP_Flag) -> Data Store Write1/1
  Data Store Read1/1 -> Chart2/2("OCP_Threshold ")
  Gain2/1 -> Gain3/1
  Gain3/1 -> Abs/1

== system PFC_69C_03_06_V01_3Phase_3_2KW/PWM Update @50KHz/Fixed Duty update_Phase_A/Archive/If Action Subsystem3/If Action Subsystem4 ==
  Action Port : ActionPort
  Data Store Read : DataStoreRead  DataStoreName=PWM_Duty_UART  IndexOptions=Index vector (dialog)  Indices=1  OutputSizes=1
  Data Store Read2 : DataStoreRead  DataStoreName=PWM_Duty_UART  IndexOptions=Index vector (dialog)  Indices=1  OutputSizes=1
  Data Store Read3 : DataStoreRead  DataStoreName=PFC_en_Phase_A  IndexOptions=Index vector (dialog)  Indices=1  OutputSizes=1
  Data Store Read4 : DataStoreRead  DataStoreName=One_Shot_Bar  IndexOptions=Index vector (dialog)  Indices=1  OutputSizes=1
  Data Store Write : DataStoreWrite  DataStoreName=PWM_DutyNearzero  IndexOptions=Index vector (dialog)  Indices=1  OutputSizes=1
  Product1 : Product  Inputs=3  OutDataTypeStr=double
  wires:
  Product1/1 -> Data Store Write/1
  Data Store Read3/1 -> Product1/1
  Data Store Read4/1 -> Product1/2
  Data Store Read2/1 -> Product1/3

== system PFC_69C_03_06_V01_3Phase_3_2KW/PWM Update @50KHz/Fixed Duty update_Phase_A/Archive/If Action Subsystem3/If Action Subsystem5 ==
  Action Port : ActionPort
  Constant : Constant  Value=100
  Data Store Read : DataStoreRead  DataStoreName=PWM_Duty_UART  IndexOptions=Index vector (dialog)  Indices=1  OutputSizes=1
  Data Store Read2 : DataStoreRead  DataStoreName=PWM_Duty_UART  IndexOptions=Index vector (dialog)  Indices=1  OutputSizes=1
  Data Store Read3 : DataStoreRead  DataStoreName=PFC_en_Phase_A  IndexOptions=Index vector (dialog)  Indices=1  OutputSizes=1
  Data Store Read4 : DataStoreRead  DataStoreName=One_Shot_Bar  IndexOptions=Index vector (dialog)  Indices=1  OutputSizes=1
  Data Store Write : DataStoreWrite  DataStoreName=PWM_DutyNearzero  IndexOptions=Index vector (dialog)  Indices=1  OutputSizes=1
  Product1 : Product  Inputs=3  OutDataTypeStr=double
  Subtract : Sum  Inputs=+-
  wires:
  Data Store Read4/1 -> Product1/2
  Data Store Read3/1 -> Product1/1
  Data Store Read2/1 -> Product1/3
  Constant/1 -> Subtract/1
  Data Store Read/1 -> Subtract/2
  Product1/1 -> Data Store Write/1

== system PFC_69C_03_06_V01_3Phase_3_2KW/PWM Update @50KHz/Fixed Duty update_Phase_B_Test/Archive/If Action Subsystem3/If Action Subsystem4 ==
  Action Port : ActionPort
  Data Store Read : DataStoreRead  DataStoreName=PWM_Duty_UART  IndexOptions=Index vector (dialog)  Indices=1  OutputSizes=1
  Data Store Read2 : DataStoreRead  DataStoreName=PWM_Duty_UART  IndexOptions=Index vector (dialog)  Indices=1  OutputSizes=1
  Data Store Read3 : DataStoreRead  DataStoreName=PFC_en_Phase_A  IndexOptions=Index vector (dialog)  Indices=1  OutputSizes=1
  Data Store Read4 : DataStoreRead  DataStoreName=One_Shot_Bar  IndexOptions=Index vector (dialog)  Indices=1  OutputSizes=1
  Data Store Write : DataStoreWrite  DataStoreName=PWM_DutyNearzero  IndexOptions=Index vector (dialog)  Indices=1  OutputSizes=1
  Product1 : Product  Inputs=3  OutDataTypeStr=double
  wires:
  Product1/1 -> Data Store Write/1
  Data Store Read3/1 -> Product1/1
  Data Store Read4/1 -> Product1/2
  Data Store Read2/1 -> Product1/3

== system PFC_69C_03_06_V01_3Phase_3_2KW/PWM Update @50KHz/Fixed Duty update_Phase_B_Test/Archive/If Action Subsystem3/If Action Subsystem5 ==
  Action Port : ActionPort
  Constant : Constant  Value=100
  Data Store Read : DataStoreRead  DataStoreName=PWM_Duty_UART  IndexOptions=Index vector (dialog)  Indices=1  OutputSizes=1
  Data Store Read2 : DataStoreRead  DataStoreName=PWM_Duty_UART  IndexOptions=Index vector (dialog)  Indices=1  OutputSizes=1
  Data Store Read3 : DataStoreRead  DataStoreName=PFC_en_Phase_A  IndexOptions=Index vector (dialog)  Indices=1  OutputSizes=1
  Data Store Read4 : DataStoreRead  DataStoreName=One_Shot_Bar  IndexOptions=Index vector (dialog)  Indices=1  OutputSizes=1
  Data Store Write : DataStoreWrite  DataStoreName=PWM_DutyNearzero  IndexOptions=Index vector (dialog)  Indices=1  OutputSizes=1
  Product1 : Product  Inputs=3  OutDataTypeStr=double
  Subtract : Sum  Inputs=+-
  wires:
  Data Store Read4/1 -> Product1/2
  Data Store Read3/1 -> Product1/1
  Data Store Read2/1 -> Product1/3
  Constant/1 -> Subtract/1
  Data Store Read/1 -> Subtract/2
  Product1/1 -> Data Store Write/1

== system PFC_69C_03_06_V01_3Phase_3_2KW/PWM Update @50KHz/Fixed Duty update_Phase_C/Archive/If Action Subsystem3/If Action Subsystem4 ==
  Action Port : ActionPort
  Data Store Read : DataStoreRead  DataStoreName=PWM_Duty_UART  IndexOptions=Index vector (dialog)  Indices=1  OutputSizes=1
  Data Store Read2 : DataStoreRead  DataStoreName=PWM_Duty_UART  IndexOptions=Index vector (dialog)  Indices=1  OutputSizes=1
  Data Store Read3 : DataStoreRead  DataStoreName=PFC_en_Phase_A  IndexOptions=Index vector (dialog)  Indices=1  OutputSizes=1
  Data Store Read4 : DataStoreRead  DataStoreName=One_Shot_Bar  IndexOptions=Index vector (dialog)  Indices=1  OutputSizes=1
  Data Store Write : DataStoreWrite  DataStoreName=PWM_DutyNearzero  IndexOptions=Index vector (dialog)  Indices=1  OutputSizes=1
  Product1 : Product  Inputs=3  OutDataTypeStr=double
  wires:
  Product1/1 -> Data Store Write/1
  Data Store Read3/1 -> Product1/1
  Data Store Read4/1 -> Product1/2
  Data Store Read2/1 -> Product1/3

== system PFC_69C_03_06_V01_3Phase_3_2KW/PWM Update @50KHz/Fixed Duty update_Phase_C/Archive/If Action Subsystem3/If Action Subsystem5 ==
  Action Port : ActionPort
  Constant : Constant  Value=100
  Data Store Read : DataStoreRead  DataStoreName=PWM_Duty_UART  IndexOptions=Index vector (dialog)  Indices=1  OutputSizes=1
  Data Store Read2 : DataStoreRead  DataStoreName=PWM_Duty_UART  IndexOptions=Index vector (dialog)  Indices=1  OutputSizes=1
  Data Store Read3 : DataStoreRead  DataStoreName=PFC_en_Phase_A  IndexOptions=Index vector (dialog)  Indices=1  OutputSizes=1
  Data Store Read4 : DataStoreRead  DataStoreName=One_Shot_Bar  IndexOptions=Index vector (dialog)  Indices=1  OutputSizes=1
  Data Store Write : DataStoreWrite  DataStoreName=PWM_DutyNearzero  IndexOptions=Index vector (dialog)  Indices=1  OutputSizes=1
  Product1 : Product  Inputs=3  OutDataTypeStr=double
  Subtract : Sum  Inputs=+-
  wires:
  Data Store Read4/1 -> Product1/2
  Data Store Read3/1 -> Product1/1
  Data Store Read2/1 -> Product1/3
  Constant/1 -> Subtract/1
  Data Store Read/1 -> Subtract/2
  Product1/1 -> Data Store Write/1

== stateflow chart PFC_69C_03_06_V01_3Phase_3_2KW/Calibration,RMS, Fault Protection @5kHz/Polarity & Near Zero check/Polarity_Near_zero_Phase_B/Chart ==
  note: 1-> Polarity -> Positive Half cycle
      | 0-> Polarity -> Negative Half cycle
  (default) -> (junction 89) : {Vabs=abs(input);}
  (junction 89) -> (junction 99) [order 1] : [input>Vref]
  (junction 89) -> (junction 103) [order 2] : {Polarity=0;}
  (junction 99) -> (junction 101) : {Polarity=1;}
  (junction 103) -> (junction 142) [order 3]
  (junction 101) -> (junction 103)
  (junction 103) -> (junction 133) [order 1] : [Near_zero==0]
      | {Count = Count+1;}
  (junction 142) -> (junction 146)
  (junction 103) -> (junction 120) [order 2] : [Vabs<VZCD_Gap]
      | {Near_zero=0;}
  (junction 133) -> (junction 120) [order 2]
  (junction 133) -> (junction 136) [order 1] : [Count>10]
      | {Near_zero=1;
      | Count=0;}
  (junction 146) -> (junction 120)
  (junction 136) -> (junction 120)
  data: input input double; Polarity output; Vabs local double =0; Vref input; VZCD_Gap input; Near_zero output double =0; Count local =0

== stateflow chart PFC_69C_03_06_V01_3Phase_3_2KW/Calibration,RMS, Fault Protection @5kHz/Relay control_corrected/Subsystem/Relay_Control1 ==
  (default) -> (junction 10)
  (junction 10) -> (junction 37) [order 2]
  (junction 37) -> (junction 40) [order 2]
  (junction 10) -> (junction 12) [order 1] : [Vin_peak_ADC>Relay_TurnON_Threshold_ADC]
  (junction 37) -> (junction 25) [order 1] : [Vin_peak_ADC<(Relay_TurnON_Threshold_ADC-5)]
  (junction 40) -> (junction 42)
  (junction 12) -> (junction 49) [order 2] : %% Relay has started.
  (junction 49) -> (junction 67) [order 1] : [PWM_Turned_on==0]
  (junction 67) -> (junction 79) [order 2]
  (junction 12) -> (junction 19) [order 1] : [Relay_Started==0]
      | {Relay_Start_Count = Relay_Start_Count + 1;}
  (junction 49) -> (junction 73) [order 2]
  (junction 67) -> (junction 68) [order 1] : [Counter_Relay > 400]
      | {
      | PWM_Turned_on=1;
      | Counter_Relay=0;
      | }
  (junction 79) -> (junction 81) : {
      | Counter_Relay = Counter_Relay + 1;
      | PWM_Turned_on=0;
      | }
  (junction 25) -> (junction 27) : [PFC_en==0]
      | {
      | Relay_Started=0;
      | Relay_Start_Count = 0;
      | PWM_Turned_on=0;
      | %% Turn off relay GPIO here
      | }
  (junction 19) -> (junction 54) [order 2]
  (junction 19) -> (junction 21) [order 1] : %%[((Vin_peak_ADC-(Vbulk_ADC_Average/2))<VIN_VBUS_DIFF)]
      | %% Vbulk is within range
  (junction 54) -> (junction 51)
  (junction 21) -> (junction 23) : [Relay_Start_Count > RELAY_START_DELAY]
      | %% waited long enough....
      |
      | {
      | Relay_Start_Count = 0;
      | Relay_Started = 1;
      | Counter_Relay=0;
      | %% Start relay GPIO here
      | }
      |
      | %% Relay started
  (junction 23) -> (junction 51)
  (junction 51) -> (junction 73)
  (junction 73) -> (junction 68)
  (junction 81) -> (junction 68)
  (junction 27) -> (junction 81)
  (junction 42) -> (junction 27)
  data: Vin_peak_ADC input; Relay_TurnON_Threshold_ADC input; RELAY_START_DELAY input; Vbulk_ADC_Average input; Relay_Start_Count local double =0; VIN_VBUS_DIFF input; PFC_en input; Relay_Started output =0; PWM_Turned_on output double =0; Counter_Relay local =0

== stateflow chart PFC_69C_03_06_V01_3Phase_3_2KW/Calibration,RMS, Fault Protection @5kHz/Fault checking/If Action Subsystem/Phase_C_Fault/Fault Check (Input OVP)_Phase_C/Chart1 ==
  (default) -> (junction 2)
  (junction 2) -> (junction 81) [order 1] : [input > Voff_Threshold]
  (junction 81) -> (junction 82) : {
      | Input_OVP_Flag=1;
      | Voff_Threshold=195;
      | }
  (junction 2) -> (junction 84) [order 2] : {
      | Input_OVP_Flag=0;
      | Voff_Threshold = 200;
      | }
  (junction 82) -> (junction 84)
  data: input input double; Input_OVP_Flag output double =0; Voff_Threshold local =200

== stateflow chart PFC_69C_03_06_V01_3Phase_3_2KW/Calibration,RMS, Fault Protection @5kHz/Fault checking/If Action Subsystem/Phase_C_Fault/Fault Check (Input UVP)_Phase_C/Chart1 ==
  (default) -> (junction 2)
  (junction 2) -> (junction 81) [order 1] : [input > Von_Threshold]
  (junction 81) -> (junction 82) : {
      | Input_UVP_Flag=0;
      | Von_Threshold=46;
      | }
  (junction 2) -> (junction 84) [order 2] : {
      | Input_UVP_Flag=1;
      | Von_Threshold = 50;
      | }
  (junction 82) -> (junction 84)
  data: input input double; Input_UVP_Flag output double =1; Von_Threshold local =50

== stateflow chart PFC_69C_03_06_V01_3Phase_3_2KW/Calibration,RMS, Fault Protection @5kHz/Fault checking/If Action Subsystem/Phase_C_Fault/Input current_OCP_Phase_C/Chart2 ==
  note: Input_in > 1A, Iin_OCP_Flag=1.
  (default) -> (junction 2)
  (junction 2) -> (junction 81) [order 1] : [input_Iin > OCP_Threshold]
  (junction 81) -> (junction 82) : {Iin_OCP_Flag=1;
      | OCP_Threshold=29;
      | }
  (junction 2) -> (junction 84) [order 2] : {Iin_OCP_Flag=0;
      | OCP_Threshold=30;}
  (junction 82) -> (junction 84)
  data: input_Iin input double; Iin_OCP_Flag output double =1; data local; OCP_Threshold input; OCP_Threshold output

== stateflow chart PFC_69C_03_06_V01_3Phase_3_2KW/Calibration,RMS, Fault Protection @5kHz/Fault checking/If Action Subsystem/PFC_en_update_Phase_C/Chart ==
  note: Local variables
      | VbusRefTemp
      | SoftStartCnt
  note: Verror = Vbulk_Ref_ADC_adjusted - Vbulk_ADC;
  (default) -> (junction 47)
  (junction 47) -> (junction 50) [order 4]
  (junction 47) -> (junction 68) [order 1] : [Vin_OVP_Flag]
  (junction 68) -> (junction 80) : {PFC_en=0;}
  (junction 47) -> (junction 15) [order 2] : [Iin_OCP_Flag]
  (junction 50) -> (junction 52) : {
      | PFC_en=1;
      | PFC_en1=1;
      | }
  (junction 47) -> (junction 5) [order 3] : [Vin_UVP_Flag]
  (junction 80) -> (junction 82)
  (junction 82) -> (junction 84)
  (junction 5) -> (junction 38) : {
      | PFC_en=0;
      | PFC_en1=0;
      | }
  (junction 15) -> (junction 20) : {PFC_en=0;
      | PFC_en1=0;}
  (junction 52) -> (junction 38)
  (junction 20) -> (junction 38)
  (junction 84) -> (junction 20)
  data: Vin_UVP_Flag input; VbusRefTemp local =0; Vin_OVP_Flag input; SoftStartCnt local =0; Vbulk_Ref_ADC_Hard_Value local =0; UVPCnt local =0; PFC_en output; PFC_en1 output; Iin_OCP_Flag input; Iin_OCP_Flag1 local
